simulink model "Ramp2_Model"  (R2023b)
settings: Solver=ode23tb  StartTime=0.0  StopTime=24  FixedStep=0.01  RelTol=1e-3
values from neighbouring files (symbols this model uses):
  BodyMass = 148+18    (= 166)    [SpiderParameters.m]
  CoverMass = 34+25+18    (= 77)    [SpiderParameters.m]
  CoxaMass = 3.1    [SpiderParameters.m]
  FemurMass = 5    [SpiderParameters.m]
  friction_force_max = mu_static * normal_force_max    [SpiderParameters.m]
  g = -9.81    [SpiderParameters.m]
  h_final = 0.020    (= 0.02)    [SpiderParameters.m]
  max_coxaRL_ang = 33*d2r    (= 0.575958653158)    [SpiderParameters.m]
  max_femurRL_ang = 60*d2r    (= 1.0471975512)    [SpiderParameters.m]
  max_tibiaRL_ang = 0 * d2r    (= 0)    [SpiderParameters.m]
  min_coxaRL_ang = -10*d2r    (= -0.174532925199)    [SpiderParameters.m]
  min_femurRL_ang = 0*d2r    (= 0)    [SpiderParameters.m]
  min_tibiaRL_ang = -60 * d2r    (= -1.0471975512)    [SpiderParameters.m]
  normal_force_max = ((total_mass)*abs(g))/4    [SpiderParameters.m]
  pitch_max = 30 * d2r    (= 0.523598775598)    [SpiderParameters.m]
  roll_max = 20* d2r    (= 0.349065850399)    [SpiderParameters.m]
  S_HoldMass = 0.275    [SpiderParameters.m]
  ServoHeadMass = 1    [SpiderParameters.m]
  ServoMass = 13    [SpiderParameters.m]
  Tf = 10    [SpiderParameters.m]
  TibiaMass = 2.8    [SpiderParameters.m]
  Ts = 0.025    [SpiderParameters.m]
  vx_max = 0.25    [SpiderParameters.m]
  vy_max = 0.25    [SpiderParameters.m]
  vz_max = 0.25    [SpiderParameters.m]
  w_max = 2*pi*60/60    (= 6.28318530718)    [SpiderParameters.m]
  y_max = 0.15    [SpiderParameters.m]
  yaw_max = 30 * d2r    (= 0.523598775598)    [SpiderParameters.m]
  z_max = 0.001* (80*cos(max_tibiaRL_ang) - 55*sin(min_femurRL_ang)-23/2)    [SpiderParameters.m]
  z_min = 0.01    [SpiderParameters.m]
undefined symbols (not defined in the file or in its folder): X, Y, Z
libraries: sm_lib x178, nesl_utility x58, simulink x2, rllib x1
(part 1 of 7)
settings Model: Creator=zaidj  LastModifiedBy=zaidj
settings DataIOCC: SaveState=on
settings DebuggingCC: MinStepSizeMsg=none
settings ModelReferenceCC: EnableRefExpFcnMdlSchedulingChecks=on
settings DiagnosticsConfigSet: SimMechanicsRigidlyBoundBlock=none
settings ExplorerConfigSet: InternalSimMechanicsExplorerSettings="<ExplorerConfiguration><canonicalview>default</canonicalview><AnimationSetting><BasePlaybackSpeed>1.0</BasePlaybackSpeed><PlaybackSpeedFactor>1.0</PlaybackSpeedFactor></AnimationSetting><TilePanel><TileInfo><Tiles Columns=\"2\" Count=\"2\" Rows=\"1\"><Column Weight=\"0.4995\"/><Column Weight=\"0.5005\"/><Row Weight=\"1\"/><Tile Height=\"1\" Width=\"1\" X=\"0\" Y=\"0\"/><Tile Height=\"1\" Width=\"1\" X=\"1\" Y=\"0\"/></Tiles></TileInfo><SceneInfo><SceneViewer><BGColor><R>0.60000002384185791</R><G>0.60000002384185791</G><B>0.60000002384185791</B></BGColor><Camera><DoPerspective>off</DoPerspective><Position><X>0.481085329227045611</X><Y>-1.63530458654059374</Y><Z>0.696778389092909234</Z></Position><Center><X>1.06087724322855692</X><Y>0.0971308355813287339</Y><Z>0.574012102480248587</Z></Center><Up><X>0.0454050290479427743</X><Y>0.0554854083698743672</Y><Z>0.997426565114035713</Z></Up><ViewLimDist>1</ViewLimDist><YLim>0.671141678199746794</YLim><XLim>0.787472902421036292</XLim></Camera></SceneViewer><SceneViewer><BGColor><R>0.60000002384185791</R><G>0.60000002384185791</G><B>0.60000002384185791</B></BGColor><Camera><DoPerspective>off</DoPerspective><Position><X>0.771557532543957647</X><Y>-0.00683193238623840994</Y><Z>1.93042042395541058</Z></Position><Center><X>0.771557532543957647</X><Y>-0.00683193238623840994</Y><Z>0.158006885579242251</Z></Center><Up><X>0</X><Y>1</Y><Z>-0</Z></Up><ViewLimDist>1</ViewLimDist><YLim>0.868793595862500712</YLim><XLim>1.02269417570100085</XLim></Camera></SceneViewer></SceneInfo></TilePanel><MechEditorPanel><Cameras/><GfxPanelCameraMap/><VideoCreator><PlaybackSpeedRatio>1.0</PlaybackSpeedRatio><FrameRate>60</FrameRate><VideoFormat>Motion JPEG AVI</VideoFormat><FrameSize>[1920 1080]</FrameSize></VideoCreator></MechEditorPanel></ExplorerConfiguration>"

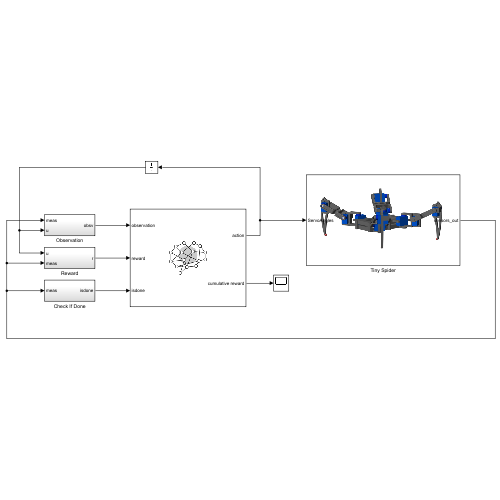
[thumbnail: Simulink's stored preview of the top-level diagram]
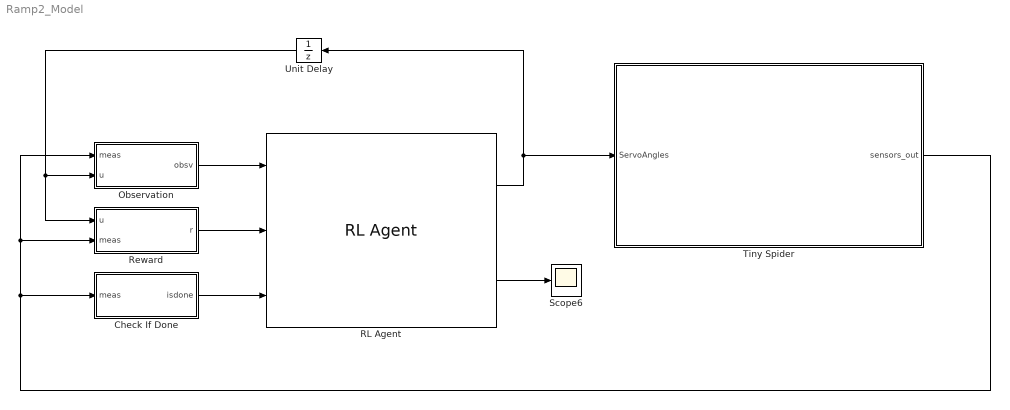
== system Ramp2_Model ==
  Check If Done : Subsystem
  Observation : Subsystem
  RL Agent : rllib/RL Agent  Agent=agent  ExternalActionAsInput=off  ProvideLastAction=off  ProvideCumRwd=on  TreatAsDirectFeedthrough=on  UseStrictObservationDataTypes=off
  Reward : Subsystem
  Scope6 : Scope
  Tiny Spider : Subsystem
      mask Display: image('$imagefile'); % Use "Edit Image" on toolstrip to change.
  Unit Delay : UnitDelay  SampleTime=-1  HasFrameUpgradeWarning=on
  wires:
  RL Agent/1 -> Tiny Spider/1(ServoAngles), Unit Delay/1
  Observation/1(obsv) -> RL Agent/1
  Reward/1(r) -> RL Agent/2
  Unit Delay/1 -> Observation/2(u), Reward/1(u)
  Check If Done/1(isdone) -> RL Agent/3
  RL Agent/2 -> Scope6/1
  Tiny Spider/1(sensors_out) -> Observation/1(meas), Reward/2(meas), Check If Done/1(meas)

== system Ramp2_Model/Check If Done ==
  note: Check if body is below minimum height
  note: Check if body angles are outside bounds
  meas : Inport
  Abs2 : Abs  ZeroCross=off  SaturateOnIntegerOverflow=off
  Bus Selector2 : BusSelector  OutputSignals=body.pos
  Compare To Constant : simulink/Logic and Bit Operations/Compare To Constant  relop=<=  const=z_min  OutDataTypeStr=boolean
  Compare To Constant2 : simulink/Logic and Bit Operations/Compare To Constant  relop=>=  const="[ roll_max  yaw_max pitch_max]"  OutDataTypeStr=boolean
  Display : Display
  Display1 : Display
  OR : Logic  Operator=OR  AllPortsSameDT=off  OutDataTypeStr=boolean
  Rate Transition : RateTransition
  Selector1 : Selector  InputPortWidth=3  IndexOptions=Index vector (dialog)  Indices=3  OutputSizes=1
  Sum of Elements2 : Sum  Inputs=+
  isdone : Outport  VectorParamsAs1DForOutWhenUnconnected=off
  wires:
  OR/1 -> Rate Transition/1
  Abs2/1 -> Display1/1, Compare To Constant2/1
  Compare To Constant2/1 -> Sum of Elements2/1
  Sum of Elements2/1 -> OR/2  "orientation criteria"
  [q2e] -> Abs2/1
  Bus Selector2/1 -> Selector1/1  "<pos>"
  Compare To Constant/1 -> OR/1  "body height criteria"
  Selector1/1 -> Display/1, Compare To Constant/1
  meas/1 -> Bus Selector2/1
  Rate Transition/1 -> isdone/1

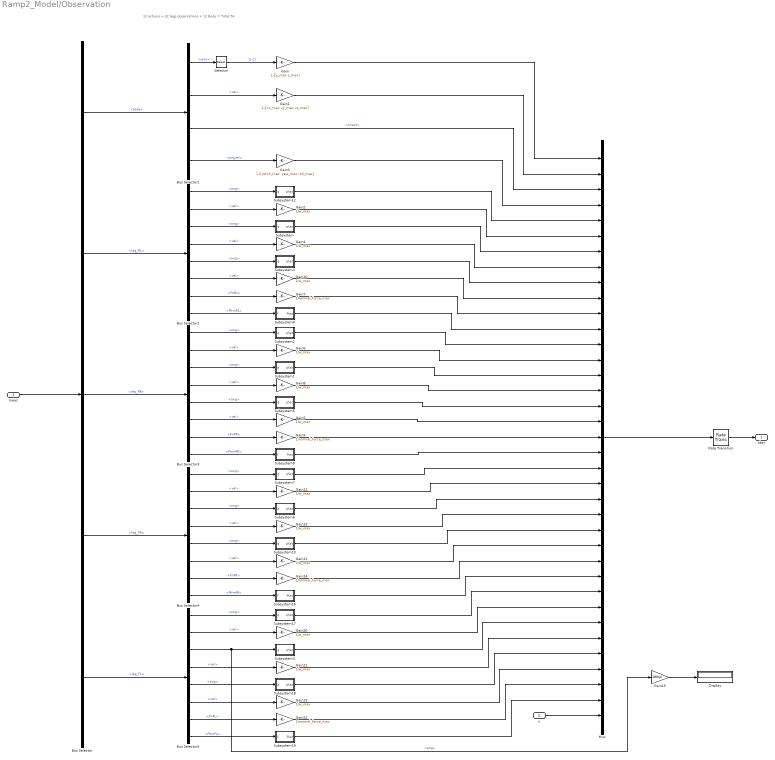
== system Ramp2_Model/Observation ==
  note: 12 actions + 32 legs observations + 12 Body = Total 56
  meas : Inport
  u : Inport  Port=2
  Bus Selector : BusSelector  OutputSignals=body,leg_RL,leg_RR,leg_FR,leg_FL
  Bus Selector1 : BusSelector  OutputSignals=pos,vel,orient,angvel
  Bus Selector2 : BusSelector  OutputSignals=RL Sensors.Tibia.ang,RL Sensors.Tibia.vel,RL Sensors.Femur.ang,RL Sensors.Femur.vel,RL Sensors.Coxa.ang,RL Sensors.Coxa.vel,FnRL,FfrmRL
  Bus Selector3 : BusSelector  OutputSignals=RR Sensor.Tibia.ang,RR Sensor.Tibia.vel,RR Sensor.Femur.ang,RR Sensor.Femur.vel,RR Sensor.Coxa.ang,RR Sensor.Coxa.vel,FnRR,FfrmRR
  Bus Selector4 : BusSelector  OutputSignals=FR sensor.Tibia.ang,FR sensor.Tibia.vel,FR sensor.Femur.ang,FR sensor.Femur.vel,FR sensor.Coxa.ang,FR sensor.Coxa.vel,FnFR,FfrmFR
  Bus Selector5 : BusSelector  OutputSignals=FL sensor.Tibia.ang,FL sensor.Tibia.vel,FL sensor.Femur.ang,FL sensor.Femur.vel,FL sensor.Coxa.ang,FL sensor.Coxa.vel,FnFL,FfrmFL
  Display : Display
  Gain : Gain  Gain=1./[y_max z_max]
  Gain1 : Gain  Gain=1./[vx_max vy_max vz_max]
  Gain{2,4..6,8,10..13,19..21} (12 alike) : Gain  Gain=1/w_max
  Gain{7,9,14,22} (4 alike) : Gain  Gain=1/normal_force_max
  Gain15 : Gain  Gain=180/pi
  Gain3 : Gain  Gain="1./[ pitch_max  yaw_max roll_max]"
  Mux : Mux  Inputs=37
  Rate Transition : RateTransition
  Selector : Selector  InputPortWidth=3  IndexOptions=Index vector (dialog)  Indices=[2 3]  OutputSizes=1
  Subsystem : Subsystem
  Subsystem1 : Subsystem
  Subsystem10 : Subsystem
  Subsystem12 : Subsystem
  Subsystem16 : Subsystem
  Subsystem17 : Subsystem
  Subsystem18 : Subsystem
  Subsystem19 : Subsystem
  Subsystem2 : Subsystem
  Subsystem3 : Subsystem
  Subsystem4 : Subsystem
  Subsystem5 : Subsystem
  Subsystem6 : Subsystem
  Subsystem7 : Subsystem
  Subsystem8 : Subsystem
  Subsystem9 : Subsystem
  obsv : Outport  VectorParamsAs1DForOutWhenUnconnected=off
  wires:
  Bus Selector1/2 -> Gain1/1  "<vel>"
  Bus Selector1/1 -> Selector/1  "<pos>"
  Mux/1 -> Rate Transition/1
  Bus Selector1/4 -> Gain3/1  "<angvel>"
  Selector/1 -> Gain/1  "[y,z]"
  meas/1 -> Bus Selector/1
  Bus Selector/1 -> Bus Selector1/1  "<body>"
  Bus Selector/2 -> Bus Selector2/1  "<leg_RL>"
  Rate Transition/1 -> obsv/1
  Bus Selector2/1 -> Subsystem12/1(q)  "<ang>"
  Bus Selector2/2 -> Gain2/1  "<vel>"
  Bus Selector2/3 -> Subsystem/1(q)  "<ang>"
  Bus Selector2/4 -> Gain4/1  "<vel>"
  Bus Selector2/5 -> Subsystem4/1(q)  "<ang>"
  Bus Selector2/6 -> Gain10/1  "<vel>"
  Bus Selector2/7 -> Gain7/1  "<FnRL>"
  Bus Selector2/8 -> Subsystem8/1(f)  "<FfrmRL>"
  Bus Selector/3 -> Bus Selector3/1  "<leg_RR>"
  Bus Selector3/4 -> Gain8/1  "<vel>"
  Bus Selector3/1 -> Subsystem2/1(q)  "<ang>"
  Bus Selector3/7 -> Gain9/1  "<FnRR>"
  Bus Selector3/2 -> Gain6/1  "<vel>"
  Bus Selector3/6 -> Gain5/1  "<vel>"
  Bus Selector3/3 -> Subsystem1/1(q)  "<ang>"
  Bus Selector3/5 -> Subsystem5/1(q)  "<ang>"
  Bus Selector3/8 -> Subsystem9/1(f)  "<FfrmRR>"
  Bus Selector/4 -> Bus Selector4/1  "<leg_FR>"
  Bus Selector4/4 -> Gain13/1  "<vel>"
  Bus Selector4/1 -> Subsystem7/1(q)  "<ang>"
  Bus Selector4/7 -> Gain14/1  "<FnFR>"
  Bus Selector4/2 -> Gain12/1  "<vel>"
  Bus Selector4/6 -> Gain11/1  "<vel>"
  Bus Selector4/3 -> Subsystem6/1(q)  "<ang>"
  Bus Selector4/5 -> Subsystem10/1(q)  "<ang>"
  Bus Selector4/8 -> Subsystem16/1(f)  "<FfrmFR>"
  Bus Selector/5 -> Bus Selector5/1  "<leg_FL>"
  Bus Selector5/4 -> Gain21/1  "<vel>"
  Bus Selector5/1 -> Subsystem17/1(q)  "<ang>"
  Bus Selector5/7 -> Gain22/1  "<FnFL>"
  Bus Selector5/2 -> Gain20/1  "<vel>"
  Bus Selector5/6 -> Gain19/1  "<vel>"
  Bus Selector5/3 -> Gain15/1, Subsystem3/1(q)  "<ang>"
  Bus Selector5/5 -> Subsystem18/1(q)  "<ang>"
  Bus Selector5/8 -> Subsystem19/1(f)  "<FfrmFL>"
  Gain/1 -> Mux/1
  Gain1/1 -> Mux/2
  Bus Selector1/3 -> Mux/3  "<orient>"
  Gain3/1 -> Mux/4
  Subsystem12/1(qhat) -> Mux/5
  Gain2/1 -> Mux/6
  Subsystem/1(qhat) -> Mux/7
  Gain4/1 -> Mux/8
  Subsystem4/1(qhat) -> Mux/9
  Gain10/1 -> Mux/10
  Gain7/1 -> Mux/11
  Subsystem8/1(fhat) -> Mux/12
  Subsystem2/1(qhat) -> Mux/13
  Gain6/1 -> Mux/14
  Subsystem1/1(qhat) -> Mux/15
  Gain8/1 -> Mux/16
  Subsystem5/1(qhat) -> Mux/17
  Gain5/1 -> Mux/18
  Gain9/1 -> Mux/19
  Subsystem9/1(fhat) -> Mux/20
  Subsystem7/1(qhat) -> Mux/21
  Gain12/1 -> Mux/22
  Subsystem6/1(qhat) -> Mux/23
  Gain13/1 -> Mux/24
  Subsystem10/1(qhat) -> Mux/25
  Gain11/1 -> Mux/26
  Gain14/1 -> Mux/27
  Subsystem16/1(fhat) -> Mux/28
  Subsystem17/1(qhat) -> Mux/29
  Gain20/1 -> Mux/30
  Subsystem3/1(qhat) -> Mux/31
  Gain21/1 -> Mux/32
  Subsystem18/1(qhat) -> Mux/33
  Gain19/1 -> Mux/34
  Gain22/1 -> Mux/35
  Subsystem19/1(fhat) -> Mux/36
  u/1 -> Mux/37
  Gain15/1 -> Display/1

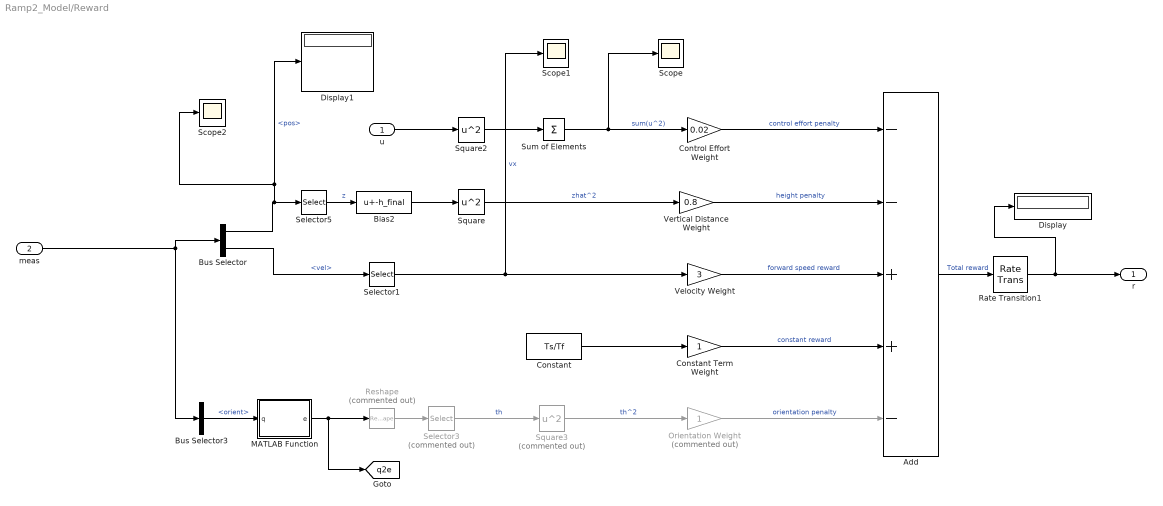
== system Ramp2_Model/Reward ==
  u : Inport
  meas : Inport  Port=2
  Add : Sum  Inputs=--++-
  Bias2 : Bias  Bias=-h_final  SaturateOnIntegerOverflow=off
  Bus Selector : BusSelector  OutputSignals=body.pos,body.vel
  Bus Selector3 : BusSelector  OutputSignals=body.orient
  "Constant " : Constant  Value=Ts/Tf  SampleTime=-1
  Constant Term Weight : Gain
  Control Effort Weight : Gain  Gain=0.02
  Display : Display
  Display1 : Display
  MATLAB Function : MATLAB Function  TreatAsAtomicUnit=on
  Orientation Weight : Gain  Commented=on
  Rate Transition1 : RateTransition
  Reshape : Reshape  Commented=on  OutputDimensions=[1]
  Scope : Scope
  Scope1 : Scope
  Scope2 : Scope
  Selector1 : Selector  InputPortWidth=3  IndexOptions=Index vector (dialog)  Indices=1  OutputSizes=1
  Selector3 : Selector  Commented=on  InputPortWidth=3  IndexOptions=Index vector (dialog)  Indices=1  OutputSizes=1
  Selector5 : Selector  InputPortWidth=3  IndexOptions=Index vector (dialog)  Indices=3  OutputSizes=1
  Square : Math  Operator=square
  Square2 : Math  Operator=square  SignedPower=on
  Square3 : Math  Commented=on  Operator=square  SignedPower=on
  Sum of Elements : Sum  Inputs=+  OutDataTypeStr=double
  Velocity Weight : Gain  Gain=3
  Vertical Distance Weight : Gain  Gain=0.8
  r : Outport  VectorParamsAs1DForOutWhenUnconnected=off
  tag scope: q2e=global
  wires:
  Selector5/1 -> Bias2/1  "z"
  Square/1 -> Vertical Distance Weight/1  "zhat^2"
  Bus Selector/2 -> Selector1/1  "<vel>"
  Sum of Elements/1 -> Scope/1, Control Effort Weight/1  "sum(u^2)"
  Bus Selector/1 -> Scope2/1, Display1/1, Selector5/1  "<pos>"
  Velocity Weight/1 -> Add/3  "forward speed reward"
  Control Effort Weight/1 -> Add/1  "control effort penalty"
  Selector1/1 -> Scope1/1, Velocity Weight/1  "vx"
  "Constant "/1 -> Constant Term Weight/1
  Square2/1 -> Sum of Elements/1
  Vertical Distance Weight/1 -> Add/2  "height penalty"
  Add/1 -> Rate Transition1/1  "Total reward"
  Bus Selector3/1 -> MATLAB Function/1(q)  "<orient>"
  Reshape/1 -> Selector3/1
  Constant Term Weight/1 -> Add/4  "constant reward"
  Orientation Weight/1 -> Add/5  "orientation penalty"
  Square3/1 -> Orientation Weight/1  "th^2"
  Selector3/1 -> Square3/1  "th"
  Bias2/1 -> Square/1
  MATLAB Function/1(e) -> [q2e], Reshape/1
  u/1 -> Square2/1
  meas/1 -> Bus Selector/1, Bus Selector3/1
  Rate Transition1/1 -> Display/1, r/1

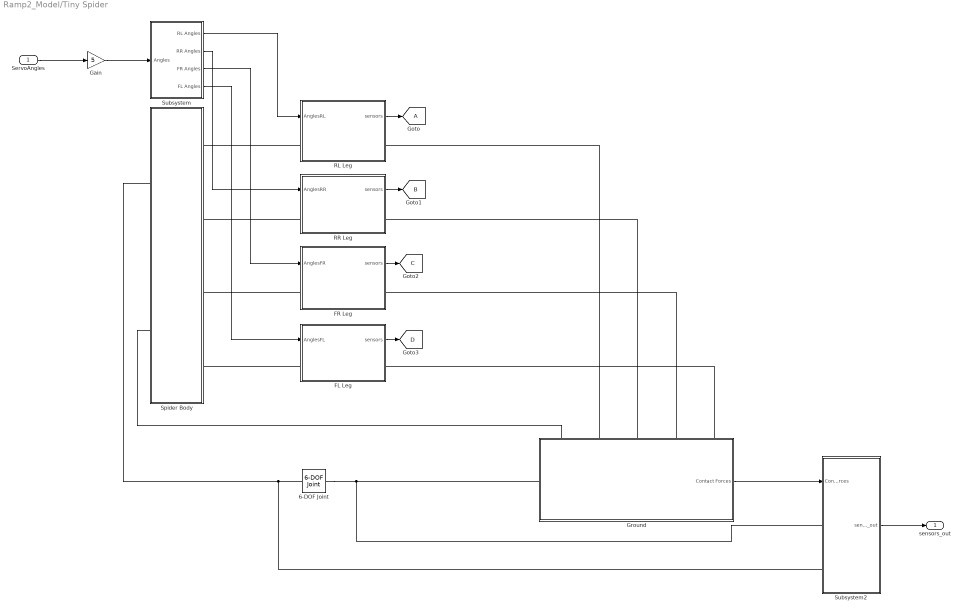
== system Ramp2_Model/Tiny Spider ==
  ServoAngles : Inport
  6-DOF Joint : sm_lib/Joints/6-DOF Joint  JointMode=Normal  SenseConstraintForce=off  SenseConstraintForceX=off  SenseConstraintForceY=off  SenseConstraintForceZ=off  SenseConstraintTorque=off  SenseConstraintTorqueX=off  SenseConstraintTorqueY=off  SenseConstraintTorqueZ=off  SenseTotalForce=off  SenseTotalForceX=off  SenseTotalForceY=off  SenseTotalForceZ=off  SenseTotalTorque=off  SenseTotalTorqueX=off  SenseTotalTorqueY=off  SenseTotalTorqueZ=off  CompositeWrenchDir=FollowerOnBase  CompositeWrenchFrame=BaseFrame  PxEquilibriumPosition=0  PxEquilibriumPositionUnits=m  PxSpringStiffness=0  PxSpringStiffnessUnits=N/m  PxDampingCoefficient=0  PxDampingCoefficientUnits=N/(m/s)  PxTorqueActuationMode=NoTorque  PxMotionActuationMode=ComputedMotion  PxSensePosition=off  PxSenseVelocity=off  PxSenseAcceleration=off  PxSenseTorqueForce=off  PxSenseLowerLimitTorqueForce=off  PxSenseUpperLimitTorqueForce=off  PxLowerLimitSpecify=off  PxLowerLimitBound=-1  PxLowerLimitBoundUnits=m  PxLowerLimitStiffness=1e6  PxLowerLimitStiffnessUnits=N/m  PxLowerLimitDamping=1e3  PxLowerLimitDampingUnits=N/(m/s)  PxLowerLimitTransitionRegionWidth=1e-4  PxLowerLimitTransitionRegionWidthUnits=m  PxUpperLimitSpecify=off  PxUpperLimitBound=1  PxUpperLimitBoundUnits=m  PxUpperLimitStiffness=1e6  PxUpperLimitStiffnessUnits=N/m  PxUpperLimitDamping=1e3  PxUpperLimitDampingUnits=N/(m/s)  PxUpperLimitTransitionRegionWidth=1e-4  PxUpperLimitTransitionRegionWidthUnits=m  PxPositionTargetSpecify=off  PxPositionTargetPriority=High  PxPositionTargetValue=0  PxPositionTargetValueUnits=m  PxVelocityTargetSpecify=on  PxVelocityTargetPriority=High  PxVelocityTargetValue=vx_init  PxVelocityTargetValueUnits=m/s  PyEquilibriumPosition=0  PyEquilibriumPositionUnits=m  PySpringStiffness=0  PySpringStiffnessUnits=N/m  PyDampingCoefficient=0  PyDampingCoefficientUnits=N/(m/s)  PyTorqueActuationMode=NoTorque  PyMotionActuationMode=ComputedMotion  PySensePosition=off  PySenseVelocity=off  PySenseAcceleration=off  PySenseTorqueForce=off  PySenseLowerLimitTorqueForce=off  PySenseUpperLimitTorqueForce=off  PyLowerLimitSpecify=off  PyLowerLimitBound=-1  PyLowerLimitBoundUnits=m  PyLowerLimitStiffness=1e6  PyLowerLimitStiffnessUnits=N/m  PyLowerLimitDamping=1e3  PyLowerLimitDampingUnits=N/(m/s)  PyLowerLimitTransitionRegionWidth=1e-4  PyLowerLimitTransitionRegionWidthUnits=m  PyUpperLimitSpecify=off  PyUpperLimitBound=1  PyUpperLimitBoundUnits=m  PyUpperLimitStiffness=1e6  PyUpperLimitStiffnessUnits=N/m  PyUpperLimitDamping=1e3  PyUpperLimitDampingUnits=N/(m/s)  PyUpperLimitTransitionRegionWidth=1e-4  PyUpperLimitTransitionRegionWidthUnits=m  PyPositionTargetSpecify=off  PyPositionTargetPriority=High  PyPositionTargetValue=70  PyPositionTargetValueUnits=mm  PyVelocityTargetSpecify=on  PyVelocityTargetPriority=High  PyVelocityTargetValue=0  PyVelocityTargetValueUnits=m/s  PzEquilibriumPosition=0  PzEquilibriumPositionUnits=mm  PzSpringStiffness=0  PzSpringStiffnessUnits=N/m  PzDampingCoefficient=0  PzDampingCoefficientUnits=N/(m/s)  PzTorqueActuationMode=NoTorque  PzMotionActuationMode=ComputedMotion  PzSensePosition=off  PzSenseVelocity=off  PzSenseAcceleration=off  PzSenseTorqueForce=off  PzSenseLowerLimitTorqueForce=off  PzSenseUpperLimitTorqueForce=off  PzLowerLimitSpecify=off  PzLowerLimitBound=-1  PzLowerLimitBoundUnits=m  PzLowerLimitStiffness=1e6  PzLowerLimitStiffnessUnits=N/m  PzLowerLimitDamping=1e3  PzLowerLimitDampingUnits=N/(m/s)  PzLowerLimitTransitionRegionWidth=1e-4  PzLowerLimitTransitionRegionWidthUnits=m  PzUpperLimitSpecify=off  PzUpperLimitBound=1  PzUpperLimitBoundUnits=m  PzUpperLimitStiffness=1e6  PzUpperLimitStiffnessUnits=N/m  PzUpperLimitDamping=1e3  PzUpperLimitDampingUnits=N/(m/s)  PzUpperLimitTransitionRegionWidth=1e-4  PzUpperLimitTransitionRegionWidthUnits=m  PzPositionTargetSpecify=on  PzPositionTargetPriority=High  PzPositionTargetValue=init_6DOF_highet  PzPositionTargetValueUnits=m  PzVelocityTargetSpecify=on  PzVelocityTargetPriority=High  PzVelocityTargetValue=vz_init  PzVelocityTargetValueUnits=m/s  SphEqPosRotationMethod=None  SphEqPosRotationAngleUnits=deg  SphEqPosRotationStandardAxis=+Z  SphEqPosRotationAngle=0.0  SphEqPosRotationArbitraryAxis=[0 0 1]  SphEqPosFollAlignAxisA=+X  SphEqPosBaseAlignAxisA=+Y  SphEqPosFollAlignAxisB=+Y  SphEqPosBaseAlignAxisB=+Z  SphEqPosRotationSequenceAxes=FollowerAxes  SphEqPosRotationSequence=XYX  SphEqPosRotationSequenceAngles=[0 0 0]  SphEqPosRotationSequenceAnglesUnits=deg  SphEqPosRotationMatrix=[1 0 0; 0 1 0; 0 0 1]  SphEqPosQuaternion=[1 0 0 0]  SphSpringStiffness=0  SphSpringStiffnessUnits=N*m/deg  SphDampingCoefficient=0  SphDampingCoefficientUnits=N*m/(deg/s)  SphActuateTorqueX=off  SphActuateTorqueY=off  SphActuateTorqueZ=off  SphActuateTorque=off  SphTorqueActuationMode=NoTorque  SphMotionActuationMode=ComputedMotion  SphActuationFrame=BaseFrame  SphSensePosition=off  SphSenseVelocityX=off  SphSenseVelocityY=off  SphSenseVelocityZ=off  SphSenseVelocity=off  SphSenseAccelerationX=off  SphSenseAccelerationY=off  SphSenseAccelerationZ=off  SphSenseAcceleration=off  SphSenseTorqueX=off  SphSenseTorqueY=off  SphSenseTorqueZ=off  SphSenseTorqueForce=off  SphSenseLowerLimitTorqueMag=off  SphSenseUpperLimitTorqueMag=off  SphSensingFrame=BaseFrame  SphLowerLimitSpecify=off  SphLowerLimitBound=15  SphLowerLimitBoundUnits=deg  SphLowerLimitStiffness=1e4  SphLowerLimitStiffnessUnits=N*m/deg  SphLowerLimitDamping=10  SphLowerLimitDampingUnits=N*m/(deg/s)  SphLowerLimitTransitionRegionWidth=0.1  SphLowerLimitTransitionRegionWidthUnits=deg  SphUpperLimitSpecify=off  SphUpperLimitBound=45  SphUpperLimitBoundUnits=deg  SphUpperLimitStiffness=1e4  SphUpperLimitStiffnessUnits=N*m/deg  SphUpperLimitDamping=10  SphUpperLimitDampingUnits=N*m/(deg/s)  SphUpperLimitTransitionRegionWidth=0.1  SphUpperLimitTransitionRegionWidthUnits=deg  SphPositionTargetRotationMethod=None  SphPositionTargetRotationAngleUnits=deg  SphPositionTargetRotationStandardAxis=+Y  SphPositionTargetRotationAngle=rampAngle  SphPositionTargetRotationArbitraryAxis=[0 0 1]  SphPositionTargetFollAlignAxisA=+X  SphPositionTargetBaseAlignAxisA=+Y  SphPositionTargetFollAlignAxisB=+Y  SphPositionTargetBaseAlignAxisB=+Z  SphPositionTargetRotationSequenceAxes=FollowerAxes  SphPositionTargetRotationSequence=XYX  SphPositionTargetRotationSequenceAngles=[0 0 0]  SphPositionTargetRotationSequenceAnglesUnits=deg  SphPositionTargetRotationMatrix=[1 0 0; 0 1 0; 0 0 1]  SphPositionTargetQuaternion=[1 0 0 0]  SphPositionTargetSpecify=off  SphPositionTargetPriority=High  SphVelocityTargetValue=[0 0 0]  SphVelocityTargetValueUnits=deg/s  SphVelocityTargetSpecify=off  SphVelocityTargetPriority=High  SphVelocityTargetInFollowerFrame=on
  FL Leg : Subsystem
      mask Display: image('$imagefile'); % Use "Edit Image" on toolstrip to change.
  FR Leg : Subsystem
      mask Display: image('$imagefile'); % Use "Edit Image" on toolstrip to change.
  Gain : Gain  Gain=5
  Goto : Goto  TagVisibility=global
  Ground : Subsystem
      settings: PortSchema="{\"entries\":[{\"content\":{\"sides\":[{\"content\":{\"connectorIds\":[\"LConn1\"]},\"type\":\"ConnectorPlacement.EquallySpacedRectSide\",\"uuid\":\"d7feb522-c0d5-44f8-966b-1947cd99c49a\"},{\"content\":{\"connectorIds\":[\"Out1\"],\"side\":\"RIGHT\"},\"type\":\"ConnectorPlacement.EquallySpacedRectSide\",\"uuid\":\"2db084ce-ae72-497d-a8f8-8ac11f652e40\"},{\"content\":{\"connectorIds\":[\"LConn2\",\"LConn3\",\"LConn4\",\"LConn5\",\"LConn6\"],\"side\":\"TOP\"},\"type\":\"ConnectorPlacement.EquallySpacedRectSide\",\"uuid\":\"6a3d0de8-411d-47e4-9d6c-3729029b09d1\"},{\"content\":{\"side\":\"BOTTOM\"},\"type\":\"ConnectorPlacement.EquallySpacedRectSide\",\"uuid\":\"d1233d80-ef3a-41f0-a5f8-137b2000161c\"}]},\"type\":\"ConnectorPlacement.EquallySpacedConnector\",\"uuid\":\"2cdc0a39-ae52-4ce6-95ca-684b3e0f786a\"}],\"packageUris\":[\"http://schema.mathworks.com/mf0/Connector/R2020b\"],\"version\":\"1.0\"}"
  RL Leg : Subsystem
      mask Display: image('$imagefile'); % Use "Edit Image" on toolstrip to change.
  RR Leg : Subsystem
      mask Display: image('$imagefile'); % Use "Edit Image" on toolstrip to change.
  Spider Body : Subsystem
  Subsystem : Subsystem
  Subsystem2 : Subsystem
  sensors_out : Outport  VectorParamsAs1DForOutWhenUnconnected=off
  tag scope: B=global, C=global, D=global
  wires:
  Ground/1("Contact Forces ") -> Subsystem2/1("Contact Forces ")
  RR Leg/1(sensors) -> [B]
  Subsystem/2(RR Angles) -> RR Leg/1(AnglesRR)
  Subsystem/3(FR Angles) -> FR Leg/1(AnglesFR)
  FL Leg/1(sensors) -> [D]
  Subsystem2/1(sensors_out) -> sensors_out/1
  Subsystem/4(FL Angles) -> FL Leg/1(AnglesFL)
  Subsystem/1(RL Angles) -> RL Leg/1(AnglesRL)
  FR Leg/1(sensors) -> [C]
  RL Leg/1(sensors) -> Goto/1
  ServoAngles/1 -> Gain/1
  Gain/1 -> Subsystem/1(Angles)
  connections:
  FL Leg/LConn1 -- Spider Body/RConn4
  RL Leg/LConn1 -- Spider Body/RConn1
  Spider Body/LConn1 -- 6-DOF Joint/RConn1 -- Subsystem2/LConn2
  Ground/LConn5 -- FR Leg/RConn1
  FR Leg/LConn1 -- Spider Body/RConn3
  Ground/LConn3 -- RL Leg/RConn1
  RR Leg/LConn1 -- Spider Body/RConn2
  Ground/LConn6 -- FL Leg/RConn1
  Subsystem2/LConn1 -- Ground/LConn1 -- 6-DOF Joint/LConn1
  Ground/LConn4 -- RR Leg/RConn1
  Spider Body/LConn2 -- Ground/LConn2

== system Ramp2_Model/Observation/Subsystem ==
  q : Inport
  Bias : Bias  Bias=-min_femurRL_ang  SaturateOnIntegerOverflow=off
  Bias1 : Bias  Bias=-1  SaturateOnIntegerOverflow=off
  Gain8 : Gain  Gain=2/(max_femurRL_ang-min_femurRL_ang)
  qhat : Outport  VectorParamsAs1DForOutWhenUnconnected=off
  wires:
  q/1 -> Bias/1
  Bias/1 -> Gain8/1
  Gain8/1 -> Bias1/1
  Bias1/1 -> qhat/1

== system Ramp2_Model/Observation/Subsystem1 ==
  q : Inport
  Bias : Bias  Bias=-(-max_femurRL_ang)  SaturateOnIntegerOverflow=off
  Bias1 : Bias  Bias=-1  SaturateOnIntegerOverflow=off
  Gain8 : Gain  Gain=2/((-min_femurRL_ang)-(-max_femurRL_ang))
  qhat : Outport  VectorParamsAs1DForOutWhenUnconnected=off
  wires:
  q/1 -> Bias/1
  Bias/1 -> Gain8/1
  Gain8/1 -> Bias1/1
  Bias1/1 -> qhat/1

== system Ramp2_Model/Observation/Subsystem10 ==
  q : Inport
  Bias : Bias  Bias=-min_coxaRL_ang  SaturateOnIntegerOverflow=off
  Bias1 : Bias  Bias=-1  SaturateOnIntegerOverflow=off
  Gain8 : Gain  Gain=2/(max_coxaRL_ang-min_coxaRL_ang)
  qhat : Outport  VectorParamsAs1DForOutWhenUnconnected=off
  wires:
  Bias1/1 -> qhat/1
  Gain8/1 -> Bias1/1
  Bias/1 -> Gain8/1
  q/1 -> Bias/1

== system Ramp2_Model/Observation/Subsystem12 ==
  q : Inport
  Bias : Bias  Bias=-min_tibiaRL_ang  SaturateOnIntegerOverflow=off
  Bias1 : Bias  Bias=-1  SaturateOnIntegerOverflow=off
  Gain8 : Gain  Gain=2/(max_tibiaRL_ang-min_tibiaRL_ang)
  qhat : Outport  VectorParamsAs1DForOutWhenUnconnected=off
  wires:
  q/1 -> Bias/1
  Bias/1 -> Gain8/1
  Gain8/1 -> Bias1/1
  Bias1/1 -> qhat/1

== system Ramp2_Model/Observation/Subsystem16 ==
  f : Inport
  Gain8 : Gain  Gain=1/friction_force_max
  Sqrt : Sqrt
  Square : Math  Operator=square  SignedPower=on
  Sum of Elements : Sum  Inputs=+
  fhat : Outport  VectorParamsAs1DForOutWhenUnconnected=off
  wires:
  f/1 -> Gain8/1
  Gain8/1 -> Square/1
  Square/1 -> Sum of Elements/1
  Sum of Elements/1 -> Sqrt/1
  Sqrt/1 -> fhat/1

== system Ramp2_Model/Observation/Subsystem17 ==
  q : Inport
  Bias : Bias  Bias=-(-max_tibiaRL_ang)  SaturateOnIntegerOverflow=off
  Bias1 : Bias  Bias=-1  SaturateOnIntegerOverflow=off
  Gain8 : Gain  Gain=2/((-min_tibiaRL_ang)-(-max_tibiaRL_ang))
  qhat : Outport  VectorParamsAs1DForOutWhenUnconnected=off
  wires:
  q/1 -> Bias/1
  Bias/1 -> Gain8/1
  Gain8/1 -> Bias1/1
  Bias1/1 -> qhat/1

== system Ramp2_Model/Observation/Subsystem18 ==
  q : Inport
  Bias : Bias  Bias=-(-max_coxaRL_ang)  SaturateOnIntegerOverflow=off
  Bias1 : Bias  Bias=-1  SaturateOnIntegerOverflow=off
  Gain8 : Gain  Gain=2/((-min_coxaRL_ang)-(-max_coxaRL_ang))
  qhat : Outport  VectorParamsAs1DForOutWhenUnconnected=off
  wires:
  Bias1/1 -> qhat/1
  Gain8/1 -> Bias1/1
  Bias/1 -> Gain8/1
  q/1 -> Bias/1

== system Ramp2_Model/Observation/Subsystem19 ==
  f : Inport
  Gain8 : Gain  Gain=1/friction_force_max
  Sqrt : Sqrt
  Square : Math  Operator=square  SignedPower=on
  Sum of Elements : Sum  Inputs=+
  fhat : Outport  VectorParamsAs1DForOutWhenUnconnected=off
  wires:
  f/1 -> Gain8/1
  Gain8/1 -> Square/1
  Square/1 -> Sum of Elements/1
  Sum of Elements/1 -> Sqrt/1
  Sqrt/1 -> fhat/1

== system Ramp2_Model/Observation/Subsystem2 ==
  q : Inport
  Bias : Bias  Bias=-(-max_tibiaRL_ang)  SaturateOnIntegerOverflow=off
  Bias1 : Bias  Bias=-1  SaturateOnIntegerOverflow=off
  Gain8 : Gain  Gain=2/((-min_tibiaRL_ang)-(-max_tibiaRL_ang))
  qhat : Outport  VectorParamsAs1DForOutWhenUnconnected=off
  wires:
  q/1 -> Bias/1
  Bias/1 -> Gain8/1
  Gain8/1 -> Bias1/1
  Bias1/1 -> qhat/1

== system Ramp2_Model/Observation/Subsystem3 ==
  q : Inport
  Bias : Bias  Bias=-(-max_femurRL_ang)  SaturateOnIntegerOverflow=off
  Bias1 : Bias  Bias=-1  SaturateOnIntegerOverflow=off
  Gain8 : Gain  Gain=2/((-min_femurRL_ang)-(-max_femurRL_ang))
  qhat : Outport  VectorParamsAs1DForOutWhenUnconnected=off
  wires:
  q/1 -> Bias/1
  Bias/1 -> Gain8/1
  Gain8/1 -> Bias1/1
  Bias1/1 -> qhat/1

== system Ramp2_Model/Observation/Subsystem4 ==
  q : Inport
  Bias : Bias  Bias=-min_coxaRL_ang  SaturateOnIntegerOverflow=off
  Bias1 : Bias  Bias=-1  SaturateOnIntegerOverflow=off
  Gain8 : Gain  Gain=2/(max_coxaRL_ang-min_coxaRL_ang)
  qhat : Outport  VectorParamsAs1DForOutWhenUnconnected=off
  wires:
  Bias1/1 -> qhat/1
  Gain8/1 -> Bias1/1
  Bias/1 -> Gain8/1
  q/1 -> Bias/1

== system Ramp2_Model/Observation/Subsystem5 ==
  q : Inport
  Bias : Bias  Bias=-(-max_coxaRL_ang)  SaturateOnIntegerOverflow=off
  Bias1 : Bias  Bias=-1  SaturateOnIntegerOverflow=off
  Gain8 : Gain  Gain=2/((-min_coxaRL_ang)-(-max_coxaRL_ang))
  qhat : Outport  VectorParamsAs1DForOutWhenUnconnected=off
  wires:
  Bias1/1 -> qhat/1
  Gain8/1 -> Bias1/1
  Bias/1 -> Gain8/1
  q/1 -> Bias/1

== system Ramp2_Model/Observation/Subsystem6 ==
  q : Inport
  Bias : Bias  Bias=-min_femurRL_ang  SaturateOnIntegerOverflow=off
  Bias1 : Bias  Bias=-1  SaturateOnIntegerOverflow=off
  Gain8 : Gain  Gain=2/(max_femurRL_ang-min_femurRL_ang)
  qhat : Outport  VectorParamsAs1DForOutWhenUnconnected=off
  wires:
  q/1 -> Bias/1
  Bias/1 -> Gain8/1
  Gain8/1 -> Bias1/1
  Bias1/1 -> qhat/1

== system Ramp2_Model/Observation/Subsystem7 ==
  q : Inport
  Bias : Bias  Bias=-min_tibiaRL_ang  SaturateOnIntegerOverflow=off
  Bias1 : Bias  Bias=-1  SaturateOnIntegerOverflow=off
  Gain8 : Gain  Gain=2/(max_tibiaRL_ang-min_tibiaRL_ang)
  qhat : Outport  VectorParamsAs1DForOutWhenUnconnected=off
  wires:
  q/1 -> Bias/1
  Bias/1 -> Gain8/1
  Gain8/1 -> Bias1/1
  Bias1/1 -> qhat/1

== system Ramp2_Model/Observation/Subsystem8 ==
  f : Inport
  Gain8 : Gain  Gain=1/friction_force_max
  Sqrt : Sqrt
  Square : Math  Operator=square  SignedPower=on
  Sum of Elements : Sum  Inputs=+
  fhat : Outport  VectorParamsAs1DForOutWhenUnconnected=off
  wires:
  f/1 -> Gain8/1
  Gain8/1 -> Square/1
  Square/1 -> Sum of Elements/1
  Sum of Elements/1 -> Sqrt/1
  Sqrt/1 -> fhat/1

== system Ramp2_Model/Observation/Subsystem9 ==
  f : Inport
  Gain8 : Gain  Gain=1/friction_force_max
  Sqrt : Sqrt
  Square : Math  Operator=square  SignedPower=on
  Sum of Elements : Sum  Inputs=+
  fhat : Outport  VectorParamsAs1DForOutWhenUnconnected=off
  wires:
  f/1 -> Gain8/1
  Gain8/1 -> Square/1
  Square/1 -> Sum of Elements/1
  Sum of Elements/1 -> Sqrt/1
  Sqrt/1 -> fhat/1
